simulink model "DCE_motor6_V2"  (R2025a)
settings: Solver=ode4  StartTime=0.0  StopTime=1  FixedStep=5e-5  RelTol=1e-3
undefined symbols (not defined in the file or in its folder): powergui
libraries: spsControlledVoltageSourceLib x24, spsControlledCurrentSourceLib x24, spsVoltageMeasurementLib x24, slpidlib x24, spspowerguiLib x2, simulink x1
(part 2 of 5)

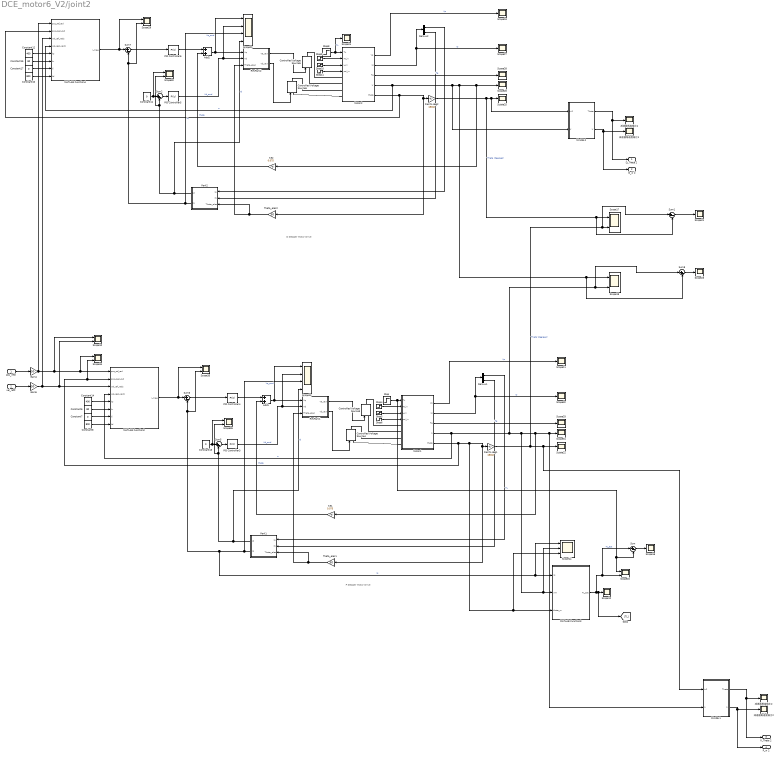
== system DCE_motor6_V2/joint2 ==
  note: D Stepper Motor Drive
  note: P Stepper Motor Drive
  pos_ref2 : Inport
  vel_ref2 : Inport  Port=2
  Add1 : Sum
  Add2 : Sum
  Constant10 : Constant  Value=800
  Constant{7,11,13,17} (4 alike) : Constant  Value=0
  Constant12 : Constant  Value=400
  Constant14 : Constant  Value=400
  Constant15 : Constant  Value=80
  Constant6 : Constant  Value=80
  Constant8 : Constant  Value=800
  Controlled Voltage Source{3..6} (4 alike) : spsControlledVoltageSourceLib/Controlled Voltage Source  Initialize=on  Source_Type=AC  Amplitude=0  Phase=0  Frequency=0  Measurements=None
  Demux1 : Demux  Outputs=2
  Demux2 : Demux  Outputs=2
  Gain4 : Gain  Gain=50
  Gain5 : Gain  Gain=50
  Ke1 : Gain  Gain=0.075
  Ke2 : Gain  Gain=0.075
  MATLAB Function2 : MATLAB Function  TreatAsAtomicUnit=on
  MATLAB Function3 : MATLAB Function  TreatAsAtomicUnit=on
  MATLAB Function4 : MATLAB Function  TreatAsAtomicUnit=on
  Mini08-1 : Subsystem
  Mini08-2 : Subsystem
  Motor1 : Subsystem
  Motor2 : Subsystem
  PID Controller{3..6} (4 alike) : slpidlib/PID Controller  Controller=PI  Form=Parallel  TimeDomain=Discrete-time  UseExternalTs=off  SampleTime=5e-5  IntegratorMethod=Forward Euler  FilterMethod=Forward Euler  ControllerParametersSource=internal  P=5  I=4000  UseKiTs=off  D=0  UseExternalDerivativeSource=off  N=100  UseFilter=on  TunerSelectOption=Transfer Function Based (PID Tuner App)  InitialConditionSource=internal  InitialConditionForIntegrator=0  InitialConditionForFilter=0  DifferentiatorICPrevScaledInput=0  ExternalReset=none  TrackingMode=off  Kt=1  LimitOutput=on  SatLimitsSource=internal  UpperSaturationLimit=24  LowerSaturationLimit=-24  LinearizeAsGain=on  AntiWindupMode=clamping  Kb=1  LimitIntegrator=on  UpperIntegratorSaturationLimit=24  LowerIntegratorSaturationLimit=-24  POutMin=[]  POutMax=[]  IOutMin=[]  IOutMax=[]  DOutMin=[]  DOutMax=[]  NOutMin=[]  NOutMax=[]  SumOutMin=[]  SumOutMax=[]  SaturationOutMin=[]  SaturationOutMax=[]  PParamMin=[]  PParamMax=[]  IParamMin=[]  IParamMax=[]  DParamMin=[]  DParamMax=[]  NParamMin=[]  NParamMax=[]  KbParamMin=[]  KbParamMax=[]  KtParamMin=[]  KtParamMax=[]  KbOutMin=[]  KbOutMax=[]  KtOutMin=[]  KtOutMax=[]  IntegratorOutMin=[]  IntegratorOutMax=[]  FilterOutMin=[]  FilterOutMax=[]  SumI1OutMin=[]  SumI1OutMax=[]  SumI2OutMin=[]  SumI2OutMax=[]  SumI3OutMin=[]  SumI3OutMax=[]  SumI4OutMin=[]  SumI4OutMax=[]  SumDOutMin=[]  SumDOutMax=[]  DifferentiatorOutMin=[]  DifferentiatorOutMax=[]  FilterDiffOutCoefMin=[]  FilterDiffOutCoefMax=[]  ReciprocalOutMin=[]  ReciprocalOutMax=[]  SumDenOutMin=[]  SumDenOutMax=[]  SumNumOutMin=[]  SumNumOutMax=[]  DivideOutMin=[]  DivideOutMax=[]  UdiffTsProdOutMin=[]  UdiffTsProdOutMax=[]  NTsProdOutMin=[]  NTsProdOutMax=[]  UintegralTsProdOutMin=[]  UintegralTsProdOutMax=[]  UngainTsProdOutMin=[]  UngainTsProdOutMax=[]  ClampingZeroOutDataTypeStr=Inherit: Inherit via back propagation  ClampingZeroOutMin=[]  ClampingZeroOutMax=[]  FilterDenConstantOutDataTypeStr=Inherit: Inherit via back propagation  FilterDenConstantOutMin=[]  FilterDenConstantOutMax=[]  PCopyOutDataTypeStr=Inherit: Inherit via back propagation  PCopyOutMin=[]  PCopyOutMax=[]  NCopyOutDataTypeStr=Inherit: Inherit via back propagation  NCopyOutMin=[]  NCopyOutMax=[]  IntegratorContinuousStateAttributes=''  IntegratorStateMustResolveToSignalObject=off  IntegratorRTWStateStorageClass=Auto  FilterContinuousStateAttributes=''  FilterStateMustResolveToSignalObject=off  FilterRTWStateStorageClass=Auto  ParallelPVariant=InternalParameters  IdealPVariant=Disabled  IVariant=InternalParameters  DVariant=Disabled  IntegratorVariant=Discrete  SatVariant=Enabled  AWVariant=DiscClampingParallel  PCopyVariant=Disabled  TRVariant=Disabled  FdbkBlocksVariant=Forward  IdealPFdbkVariant=Disabled  SatFdbkVariant=Disabled  DerivativeFilterVariant=Disabled  NVariant=Disabled  NCopyVariant=Disabled_SignalSpec  FilterICVariant=Disabled  IntegratorICVariant=InternalICs  ExternalResetVariant=Disabled  TRSumVariant=Passthrough  SumFdbkVariant=Disabled  SumVariant=Sum_PI  TsampFilterVariant=InternalTs  TsampNgainVariant=Passthrough  TsampIntegralVariant=Disabled_SignalSpec  ExternalSaturationOutDataTypeStr=Inherit: Same as second input  DerivativeSourceVariant=Disabled  PreIntVariant=InternalPreInt
  Park1 : MATLAB Function  TreatAsAtomicUnit=on
  Park2 : MATLAB Function  TreatAsAtomicUnit=on
  Rad to deg1 : Gain  Gain=180/pi
  Rad to deg2 : Gain  Gain=180/pi
  RevPark1 : MATLAB Function  TreatAsAtomicUnit=on
  RevPark2 : MATLAB Function  TreatAsAtomicUnit=on
  Scope{10,15,17,19,29..30,34..36} (9 alike) : Scope  NumInputPorts=2
      Scope10 settings: ActiveDisplayYMinimum=-5.2481835137744008  ActiveDisplayYMaximum=47.233651623969614  DataLoggingVariableName=ScopeData27
      Scope15 settings: ActiveDisplayYMinimum=0.0075000000000000006  ActiveDisplayYMaximum=0.0325  DataLoggingVariableName=ScopeData34
      Scope17 settings: ActiveDisplayYMinimum=1363.1836491868808  ActiveDisplayYMaximum=1375.04702581976  DataLoggingVariableName=ScopeData36
      Scope19 settings: ActiveDisplayYMinimum=-9.7785388194430141  ActiveDisplayYMaximum=52.407441398347267  DataLoggingVariableName=ScopeData38
      Scope29 settings: ActiveDisplayYMinimum=-0.018504547079538081  ActiveDisplayYMaximum=0.49853620070628168  DataLoggingVariableName=ScopeData28
      Scope30 settings: ActiveDisplayYMinimum=-0.068250226127922337  ActiveDisplayYMaximum=0.064256506451961737  DataLoggingVariableName=ScopeData29
      Scope34 settings: ActiveDisplayYMinimum=-10.860061692792559  ActiveDisplayYMaximum=61.442988659524922  DataLoggingVariableName=ScopeData49
      Scope35 settings: ActiveDisplayYMinimum=-0.018504547079538081  ActiveDisplayYMaximum=0.49853620070628168  DataLoggingVariableName=ScopeData50
      Scope36 settings: ActiveDisplayYMinimum=-0.068250226127922337  ActiveDisplayYMaximum=0.064256506451961737  DataLoggingVariableName=ScopeData51
  Scope{11..12,16,18,21..28,31..33} (15 alike) : Scope
      Scope11 settings: ActiveDisplayYMinimum=-19.096901402816375  ActiveDisplayYMaximum=19.120590576315788  DataLoggingVariableName=ScopeData30
      Scope12 settings: ActiveDisplayYMinimum=0.0055558714492785766  ActiveDisplayYMaximum=0.04791549784383016  DataLoggingVariableName=ScopeData31
      Scope16 settings: ActiveDisplayYMinimum=-0.00045623090907525666  ActiveDisplayYMaximum=0.00044225246132360179  DataLoggingVariableName=ScopeData35
      Scope18 settings: ActiveDisplayYMinimum=-19.096901402816375  ActiveDisplayYMaximum=19.120590576315788  DataLoggingVariableName=ScopeData37
      Scope21 settings: ActiveDisplayYMinimum=-9.08103109878298  ActiveDisplayYMaximum=1.6684669955642857  DataLoggingVariableName=ScopeData40
      Scope22 settings: ActiveDisplayYMinimum=-70.559876705932709  ActiveDisplayYMaximum=631.53921004933659  DataLoggingVariableName=ScopeData41
      Scope23 settings: ActiveDisplayYMinimum=-1.5635296954169715  ActiveDisplayYMaximum=0.72593411203052016  DataLoggingVariableName=ScopeData42
      Scope24 settings: ActiveDisplayYMinimum=-0.0062150346375224163  ActiveDisplayYMaximum=0.055935311737701762  DataLoggingVariableName=ScopeData43
      Scope25 settings: ActiveDisplayYMinimum=-70.559876705932709  ActiveDisplayYMaximum=631.53921004933659  DataLoggingVariableName=ScopeData44
      Scope26 settings: ActiveDisplayYMinimum=-452.6835395386438  ActiveDisplayYMaximum=318.93705127381384  DataLoggingVariableName=ScopeData45
      Scope27 settings: ActiveDisplayYMinimum=-0.40449771436693455  ActiveDisplayYMaximum=0.64067173662257559  DataLoggingVariableName=ScopeData25
      Scope28 settings: ActiveDisplayYMinimum=-0.046646220623980633  ActiveDisplayYMaximum=0.10063848186154864  DataLoggingVariableName=ScopeData26
      Scope31 settings: ActiveDisplayYMinimum=-115.17645332437448  ActiveDisplayYMaximum=118.37044346456712  DataLoggingVariableName=ScopeData46
      Scope32 settings: ActiveDisplayYMinimum=-0.40449771436693455  ActiveDisplayYMaximum=0.64067173662257559  DataLoggingVariableName=ScopeData47
      Scope33 settings: ActiveDisplayYMinimum=-0.046646220623980633  ActiveDisplayYMaximum=0.10063848186154864  DataLoggingVariableName=ScopeData48
  Scope13 : Scope  NumInputPorts=4
      settings: ActiveDisplayYMinimum=-0.68813129304418319  ActiveDisplayYMaximum=6.2555990509558841  DataLoggingVariableName=ScopeData32
  Scope14 : Scope  NumInputPorts=3
      settings: ActiveDisplayYMinimum=-0.052783691584462819  ActiveDisplayYMaximum=0.4750532242601655  DataLoggingVariableName=ScopeData33
  Scope20 : Scope  NumInputPorts=4
      settings: ActiveDisplayYMinimum=-0.68813129304418319  ActiveDisplayYMaximum=6.2555990509558841  DataLoggingVariableName=ScopeData39
  Step : Step  Time=0  Before=0.01  After=0.01  SampleTime=0
  Step10 : Step  Time=0  Before=0.00544  After=0.00544  SampleTime=0
  Step11 : Step  Time=0  Before=0.0015  After=0.0015  SampleTime=0
  Step4 : Step  Time=0  Before=4.85  After=4.85  SampleTime=0
  Step5 : Step  Time=0  Before=0.00544  After=0.00544  SampleTime=0
  Step6 : Step  Time=0  Before=0.0015  After=0.0015  SampleTime=0
  Step8 : Step  Time=0  Before=0.01  After=0.01  SampleTime=0
  Step9 : Step  Time=0  Before=4.85  After=4.85  SampleTime=0
  Sum{,1..2,5..8} (7 alike) : Sum  Inputs=|+-
  Theta_elec1 : Gain  Gain=50
  Theta_elec2 : Gain  Gain=50
  减速器角度输出1 : Scope
      settings: ActiveDisplayYMinimum=-3.2575204385667078  ActiveDisplayYMaximum=25.318176358378867  DataLoggingVariableName=ScopeData53
  减速器角度输出2 : Scope
      settings: ActiveDisplayYMinimum=-3.2575204385667078  ActiveDisplayYMaximum=25.318176358378867  DataLoggingVariableName=ScopeData56
  减速器角速度输出1 : Scope
      settings: ActiveDisplayYMinimum=-0.049701649268213327  ActiveDisplayYMaximum=0.44324985732957672  DataLoggingVariableName=ScopeData54
  减速器角速度输出2 : Scope
      settings: ActiveDisplayYMinimum=-0.049701649268213327  ActiveDisplayYMaximum=0.44324985732957672  DataLoggingVariableName=ScopeData57
  D_Theta 2 : Outport
  D_w 2 : Outport  Port=2
  P_Theta 2 : Outport  Port=3
  P_w 2 : Outport  Port=4
  wires:
  Sum8/1 -> Scope23/1
  Sum1/1 -> Scope21/1
  Step8/1 -> Scope24/1, Motor2/1(TL)  "TL"
  Motor2/1(Vp) -> Scope18/1  "Vp"
  Motor2/2(Ip) -> Demux2/1, Scope27/1  "Ip"
  Park2/2(Iq) -> Scope20/3, Scope29/2, Sum7/2  "Iq"
  Park2/1(Id) -> Scope20/4, Scope30/2, Sum2/2  "Id"
  Constant11/1 -> Scope30/1, Sum2/1
  PID Controller6/1 -> Add2/1
  MATLAB Function4/1(I_mag) -> Scope29/1, Sum7/1
  Demux2/1 -> Park2/1(Ia)
  Sum7/1 -> PID Controller6/1
  Motor2/5(theta) -> MATLAB Function4/2(pos_real_rad), Rad to deg2/1, Theta_elec2/1  "theta"
  Constant12/1 -> MATLAB Function4/5(kp)
  Sum2/1 -> PID Controller5/1
  Step10/1 -> Motor2/3(L_in)
  Ke2/1 -> Add2/2
  Motor2/3(Te) -> Scope28/1  "Te"
  RevPark2/2(Vb_raw) -> Controlled Voltage Source6/1
  Step11/1 -> Motor2/4(psi_in)
  Theta_elec2/1 -> RevPark2/3(Theta_elec), Park2/3(Theta_elec)
  Constant17/1 -> MATLAB Function4/7(ki)
  Add2/1 -> Scope20/1, RevPark2/1(Vq)  "Vq_cmd"
  PID Controller5/1 -> Scope20/2, RevPark2/2(Vd)  "Vd_cmd"
  Step/1 -> Sum/2, Scope15/1, Motor1/1(TL)  "TL"
  Motor2/4(w) -> MATLAB Function4/4(vel_real_rads), Mini08-2/2(w), Sum8/2, Scope19/1, Ke2/1, Scope26/1  "w"
  MATLAB Function3/1(TL_est) -> Sum/1, Scope15/2, [TL], Scope12/1  "TL_est"
  Sum/1 -> Scope16/1
  PID Controller3/1 -> Scope13/2, RevPark1/2(Vd)  "Vd_cmd"
  Motor1/4(w) -> MATLAB Function2/4(vel_real_rads), Sum8/1, Scope19/2, Scope14/2, MATLAB Function3/2(wm), Ke1/1, Mini08-1/2(w), Scope31/1  "w"
  Step9/1 -> Motor2/2(IR_in)
  Add1/1 -> Scope13/1, RevPark1/1(Vq)  "Vq_cmd"
  Constant14/1 -> MATLAB Function2/5(kp)
  Park1/1(Id) -> Scope13/4, Scope36/2, Sum5/2  "Id"
  Constant6/1 -> MATLAB Function2/6(kv)
  Constant15/1 -> MATLAB Function4/6(kv)
  Constant7/1 -> MATLAB Function2/7(ki)
  Theta_elec1/1 -> RevPark1/3(Theta_elec), Park1/3(Theta_elec)
  Motor1/5(theta) -> Scope34/2, MATLAB Function2/2(pos_real_rad), Scope14/3, MATLAB Function3/3(theta_m), Rad to deg1/1, Theta_elec1/1  "theta"
  Sum5/1 -> PID Controller3/1
  Step5/1 -> Motor1/3(L_in)
  Ke1/1 -> Add1/2
  Step6/1 -> Motor1/4(psi_in)
  Sum6/1 -> PID Controller4/1
  Rad to deg1/1 -> Sum1/1, Scope17/2, Mini08-1/1(In2), Scope22/1  "Theta (degrees)"
  RevPark1/2(Vb_raw) -> Controlled Voltage Source4/1
  Demux2/2 -> Park2/2(Ib)
  Motor1/3(Te) -> Scope33/1  "Te"
  Rad to deg2/1 -> Sum1/2, Scope17/1, Mini08-2/1(In2), Scope25/1  "Theta (degrees)"
  RevPark1/1(Va_raw) -> Controlled Voltage Source3/1
  Constant8/1 -> MATLAB Function2/8(kd)
  Demux1/1 -> Park1/1(Ia)
  Motor1/1(Vp) -> Scope11/1  "Vp"
  RevPark2/1(Va_raw) -> Controlled Voltage Source5/1
  Step4/1 -> Motor1/2(IR_in)
  Park1/2(Iq) -> Scope13/3, Scope14/1, MATLAB Function3/1(iq), Scope35/2, Sum6/2  "Iq"
  Constant10/1 -> MATLAB Function4/8(kd)
  MATLAB Function2/1(I_mag) -> Scope35/1, Sum6/1
  Motor1/2(Ip) -> Demux1/1, Scope32/1  "Ip"
  Constant13/1 -> Scope36/1, Sum5/1
  PID Controller4/1 -> Add1/1
  Demux1/2 -> Park1/2(Ib)
  vel_ref2/1 -> Gain5/1
  Gain4/1 -> Scope10/1, Scope34/1, MATLAB Function2/1(pos_ref_rad), MATLAB Function4/1(pos_ref_rad)
  pos_ref2/1 -> Gain4/1
  Gain5/1 -> Scope10/2, MATLAB Function2/3(vel_ref_rads), MATLAB Function4/3(vel_ref_rads)
  Mini08-2/1("Theta ") -> D_Theta 2/1, 减速器角度输出1/1
  Mini08-2/2("w ") -> D_w 2/1, 减速器角速度输出1/1
  Mini08-1/2("w ") -> P_w 2/1, 减速器角速度输出2/1
  Mini08-1/1("Theta ") -> P_Theta 2/1, 减速器角度输出2/1
  connections:
  Motor1/LConn4 -- Controlled Voltage Source4/LConn1
  Motor2/LConn4 -- Controlled Voltage Source6/LConn1
  Motor1/LConn2 -- Controlled Voltage Source3/LConn1
  Motor2/LConn1 -- Controlled Voltage Source5/RConn1
  Motor1/LConn1 -- Controlled Voltage Source3/RConn1
  Motor2/LConn2 -- Controlled Voltage Source5/LConn1
  Motor1/LConn3 -- Controlled Voltage Source4/RConn1
  Motor2/LConn3 -- Controlled Voltage Source6/RConn1

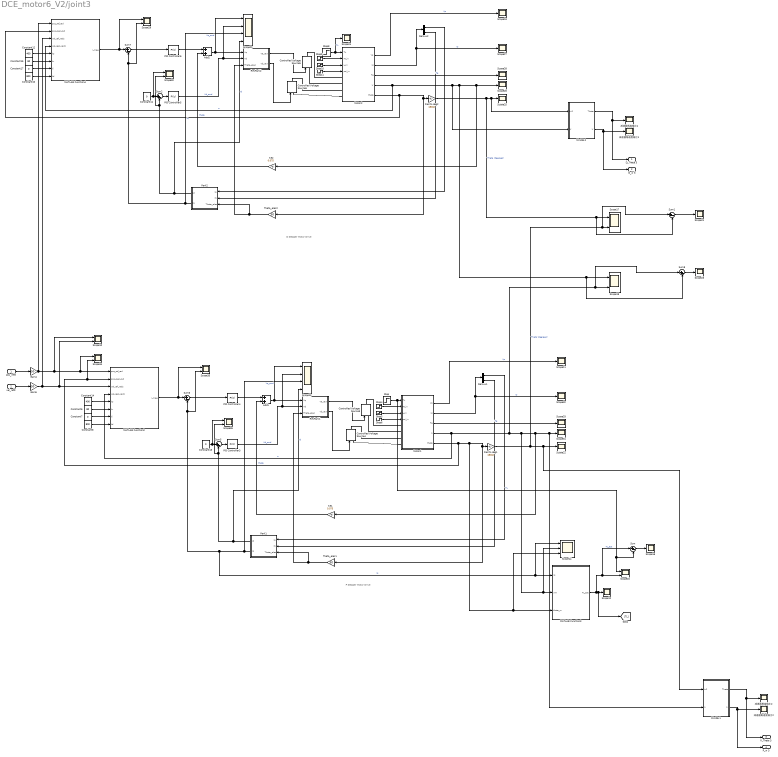
== system DCE_motor6_V2/joint3 ==
  note: D Stepper Motor Drive
  note: P Stepper Motor Drive
  pos_ref3 : Inport
  vel_ref3 : Inport  Port=2
  Add1 : Sum
  Add2 : Sum
  Constant10 : Constant  Value=800
  Constant{7,11,13,17} (4 alike) : Constant  Value=0
  Constant12 : Constant  Value=400
  Constant14 : Constant  Value=400
  Constant15 : Constant  Value=80
  Constant6 : Constant  Value=80
  Constant8 : Constant  Value=800
  Controlled Voltage Source{3..6} (4 alike) : spsControlledVoltageSourceLib/Controlled Voltage Source  Initialize=on  Source_Type=AC  Amplitude=0  Phase=0  Frequency=0  Measurements=None
  Demux1 : Demux  Outputs=2
  Demux2 : Demux  Outputs=2
  Gain4 : Gain  Gain=50
  Gain5 : Gain  Gain=50
  Ke1 : Gain  Gain=0.075
  Ke2 : Gain  Gain=0.075
  MATLAB Function2 : MATLAB Function  TreatAsAtomicUnit=on
  MATLAB Function3 : MATLAB Function  TreatAsAtomicUnit=on
  MATLAB Function4 : MATLAB Function  TreatAsAtomicUnit=on
  Mini08-1 : Subsystem
  Mini08-2 : Subsystem
  Motor1 : Subsystem
  Motor2 : Subsystem
  PID Controller{3..6} (4 alike) : slpidlib/PID Controller  Controller=PI  Form=Parallel  TimeDomain=Discrete-time  UseExternalTs=off  SampleTime=5e-5  IntegratorMethod=Forward Euler  FilterMethod=Forward Euler  ControllerParametersSource=internal  P=5  I=4000  UseKiTs=off  D=0  UseExternalDerivativeSource=off  N=100  UseFilter=on  TunerSelectOption=Transfer Function Based (PID Tuner App)  InitialConditionSource=internal  InitialConditionForIntegrator=0  InitialConditionForFilter=0  DifferentiatorICPrevScaledInput=0  ExternalReset=none  TrackingMode=off  Kt=1  LimitOutput=on  SatLimitsSource=internal  UpperSaturationLimit=24  LowerSaturationLimit=-24  LinearizeAsGain=on  AntiWindupMode=clamping  Kb=1  LimitIntegrator=on  UpperIntegratorSaturationLimit=24  LowerIntegratorSaturationLimit=-24  POutMin=[]  POutMax=[]  IOutMin=[]  IOutMax=[]  DOutMin=[]  DOutMax=[]  NOutMin=[]  NOutMax=[]  SumOutMin=[]  SumOutMax=[]  SaturationOutMin=[]  SaturationOutMax=[]  PParamMin=[]  PParamMax=[]  IParamMin=[]  IParamMax=[]  DParamMin=[]  DParamMax=[]  NParamMin=[]  NParamMax=[]  KbParamMin=[]  KbParamMax=[]  KtParamMin=[]  KtParamMax=[]  KbOutMin=[]  KbOutMax=[]  KtOutMin=[]  KtOutMax=[]  IntegratorOutMin=[]  IntegratorOutMax=[]  FilterOutMin=[]  FilterOutMax=[]  SumI1OutMin=[]  SumI1OutMax=[]  SumI2OutMin=[]  SumI2OutMax=[]  SumI3OutMin=[]  SumI3OutMax=[]  SumI4OutMin=[]  SumI4OutMax=[]  SumDOutMin=[]  SumDOutMax=[]  DifferentiatorOutMin=[]  DifferentiatorOutMax=[]  FilterDiffOutCoefMin=[]  FilterDiffOutCoefMax=[]  ReciprocalOutMin=[]  ReciprocalOutMax=[]  SumDenOutMin=[]  SumDenOutMax=[]  SumNumOutMin=[]  SumNumOutMax=[]  DivideOutMin=[]  DivideOutMax=[]  UdiffTsProdOutMin=[]  UdiffTsProdOutMax=[]  NTsProdOutMin=[]  NTsProdOutMax=[]  UintegralTsProdOutMin=[]  UintegralTsProdOutMax=[]  UngainTsProdOutMin=[]  UngainTsProdOutMax=[]  ClampingZeroOutDataTypeStr=Inherit: Inherit via back propagation  ClampingZeroOutMin=[]  ClampingZeroOutMax=[]  FilterDenConstantOutDataTypeStr=Inherit: Inherit via back propagation  FilterDenConstantOutMin=[]  FilterDenConstantOutMax=[]  PCopyOutDataTypeStr=Inherit: Inherit via back propagation  PCopyOutMin=[]  PCopyOutMax=[]  NCopyOutDataTypeStr=Inherit: Inherit via back propagation  NCopyOutMin=[]  NCopyOutMax=[]  IntegratorContinuousStateAttributes=''  IntegratorStateMustResolveToSignalObject=off  IntegratorRTWStateStorageClass=Auto  FilterContinuousStateAttributes=''  FilterStateMustResolveToSignalObject=off  FilterRTWStateStorageClass=Auto  ParallelPVariant=InternalParameters  IdealPVariant=Disabled  IVariant=InternalParameters  DVariant=Disabled  IntegratorVariant=Discrete  SatVariant=Enabled  AWVariant=DiscClampingParallel  PCopyVariant=Disabled  TRVariant=Disabled  FdbkBlocksVariant=Forward  IdealPFdbkVariant=Disabled  SatFdbkVariant=Disabled  DerivativeFilterVariant=Disabled  NVariant=Disabled  NCopyVariant=Disabled_SignalSpec  FilterICVariant=Disabled  IntegratorICVariant=InternalICs  ExternalResetVariant=Disabled  TRSumVariant=Passthrough  SumFdbkVariant=Disabled  SumVariant=Sum_PI  TsampFilterVariant=InternalTs  TsampNgainVariant=Passthrough  TsampIntegralVariant=Disabled_SignalSpec  ExternalSaturationOutDataTypeStr=Inherit: Same as second input  DerivativeSourceVariant=Disabled  PreIntVariant=InternalPreInt
  Park1 : MATLAB Function  TreatAsAtomicUnit=on
  Park2 : MATLAB Function  TreatAsAtomicUnit=on
  Rad to deg1 : Gain  Gain=180/pi
  Rad to deg2 : Gain  Gain=180/pi
  RevPark1 : MATLAB Function  TreatAsAtomicUnit=on
  RevPark2 : MATLAB Function  TreatAsAtomicUnit=on
  Scope{10,15,17,19,29..30,34..36} (9 alike) : Scope  NumInputPorts=2
      Scope10 settings: ActiveDisplayYMinimum=-5.2481835137744008  ActiveDisplayYMaximum=47.233651623969614  DataLoggingVariableName=ScopeData27
      Scope15 settings: ActiveDisplayYMinimum=0.0075000000000000006  ActiveDisplayYMaximum=0.0325  DataLoggingVariableName=ScopeData34
      Scope17 settings: ActiveDisplayYMinimum=1363.1836491868808  ActiveDisplayYMaximum=1375.04702581976  DataLoggingVariableName=ScopeData36
      Scope19 settings: ActiveDisplayYMinimum=-9.7785388194430141  ActiveDisplayYMaximum=52.407441398347267  DataLoggingVariableName=ScopeData38
      Scope29 settings: ActiveDisplayYMinimum=-0.018504547079538081  ActiveDisplayYMaximum=0.49853620070628168  DataLoggingVariableName=ScopeData28
      Scope30 settings: ActiveDisplayYMinimum=-0.068250226127922337  ActiveDisplayYMaximum=0.064256506451961737  DataLoggingVariableName=ScopeData29
      Scope34 settings: ActiveDisplayYMinimum=-10.860061692792559  ActiveDisplayYMaximum=61.442988659524922  DataLoggingVariableName=ScopeData49
      Scope35 settings: ActiveDisplayYMinimum=-0.018504547079538081  ActiveDisplayYMaximum=0.49853620070628168  DataLoggingVariableName=ScopeData50
      Scope36 settings: ActiveDisplayYMinimum=-0.068250226127922337  ActiveDisplayYMaximum=0.064256506451961737  DataLoggingVariableName=ScopeData51
  Scope{11..12,16,18,21..28,31..33} (15 alike) : Scope
      Scope11 settings: ActiveDisplayYMinimum=-19.096901402816375  ActiveDisplayYMaximum=19.120590576315788  DataLoggingVariableName=ScopeData30
      Scope12 settings: ActiveDisplayYMinimum=0.0055558714492785766  ActiveDisplayYMaximum=0.04791549784383016  DataLoggingVariableName=ScopeData31
      Scope16 settings: ActiveDisplayYMinimum=-0.00045623090907525666  ActiveDisplayYMaximum=0.00044225246132360179  DataLoggingVariableName=ScopeData35
      Scope18 settings: ActiveDisplayYMinimum=-19.096901402816375  ActiveDisplayYMaximum=19.120590576315788  DataLoggingVariableName=ScopeData37
      Scope21 settings: ActiveDisplayYMinimum=-9.08103109878298  ActiveDisplayYMaximum=1.6684669955642857  DataLoggingVariableName=ScopeData40
      Scope22 settings: ActiveDisplayYMinimum=-70.559876705932709  ActiveDisplayYMaximum=631.53921004933659  DataLoggingVariableName=ScopeData41
      Scope23 settings: ActiveDisplayYMinimum=-1.5635296954169715  ActiveDisplayYMaximum=0.72593411203052016  DataLoggingVariableName=ScopeData42
      Scope24 settings: ActiveDisplayYMinimum=-0.0062150346375224163  ActiveDisplayYMaximum=0.055935311737701762  DataLoggingVariableName=ScopeData43
      Scope25 settings: ActiveDisplayYMinimum=-70.559876705932709  ActiveDisplayYMaximum=631.53921004933659  DataLoggingVariableName=ScopeData44
      Scope26 settings: ActiveDisplayYMinimum=-452.6835395386438  ActiveDisplayYMaximum=318.93705127381384  DataLoggingVariableName=ScopeData45
      Scope27 settings: ActiveDisplayYMinimum=-0.40449771436693455  ActiveDisplayYMaximum=0.64067173662257559  DataLoggingVariableName=ScopeData25
      Scope28 settings: ActiveDisplayYMinimum=-0.046646220623980633  ActiveDisplayYMaximum=0.10063848186154864  DataLoggingVariableName=ScopeData26
      Scope31 settings: ActiveDisplayYMinimum=-115.17645332437448  ActiveDisplayYMaximum=118.37044346456712  DataLoggingVariableName=ScopeData46
      Scope32 settings: ActiveDisplayYMinimum=-0.40449771436693455  ActiveDisplayYMaximum=0.64067173662257559  DataLoggingVariableName=ScopeData47
      Scope33 settings: ActiveDisplayYMinimum=-0.046646220623980633  ActiveDisplayYMaximum=0.10063848186154864  DataLoggingVariableName=ScopeData48
  Scope13 : Scope  NumInputPorts=4
      settings: ActiveDisplayYMinimum=-0.68813129304418319  ActiveDisplayYMaximum=6.2555990509558841  DataLoggingVariableName=ScopeData32
  Scope14 : Scope  NumInputPorts=3
      settings: ActiveDisplayYMinimum=-0.052783691584462819  ActiveDisplayYMaximum=0.4750532242601655  DataLoggingVariableName=ScopeData33
  Scope20 : Scope  NumInputPorts=4
      settings: ActiveDisplayYMinimum=-0.68813129304418319  ActiveDisplayYMaximum=6.2555990509558841  DataLoggingVariableName=ScopeData39
  Step : Step  Time=0  Before=0.01  After=0.01  SampleTime=0
  Step10 : Step  Time=0  Before=0.00544  After=0.00544  SampleTime=0
  Step11 : Step  Time=0  Before=0.0015  After=0.0015  SampleTime=0
  Step4 : Step  Time=0  Before=4.85  After=4.85  SampleTime=0
  Step5 : Step  Time=0  Before=0.00544  After=0.00544  SampleTime=0
  Step6 : Step  Time=0  Before=0.0015  After=0.0015  SampleTime=0
  Step8 : Step  Time=0  Before=0.01  After=0.01  SampleTime=0
  Step9 : Step  Time=0  Before=4.85  After=4.85  SampleTime=0
  Sum{,1..2,5..8} (7 alike) : Sum  Inputs=|+-
  Theta_elec1 : Gain  Gain=50
  Theta_elec2 : Gain  Gain=50
  减速器角度输出1 : Scope
      settings: ActiveDisplayYMinimum=-3.2575204385667078  ActiveDisplayYMaximum=25.318176358378867  DataLoggingVariableName=ScopeData53
  减速器角度输出2 : Scope
      settings: ActiveDisplayYMinimum=-3.2575204385667078  ActiveDisplayYMaximum=25.318176358378867  DataLoggingVariableName=ScopeData56
  减速器角速度输出1 : Scope
      settings: ActiveDisplayYMinimum=-0.049701649268213327  ActiveDisplayYMaximum=0.44324985732957672  DataLoggingVariableName=ScopeData54
  减速器角速度输出2 : Scope
      settings: ActiveDisplayYMinimum=-0.049701649268213327  ActiveDisplayYMaximum=0.44324985732957672  DataLoggingVariableName=ScopeData57
  D_Theta 3 : Outport
  D_w 3 : Outport  Port=2
  P_Theta 3 : Outport  Port=3
  P_w 3 : Outport  Port=4
  wires:
  Sum8/1 -> Scope23/1
  Sum1/1 -> Scope21/1
  Step8/1 -> Scope24/1, Motor2/1(TL)  "TL"
  Motor2/1(Vp) -> Scope18/1  "Vp"
  Motor2/2(Ip) -> Demux2/1, Scope27/1  "Ip"
  Park2/2(Iq) -> Scope20/3, Scope29/2, Sum7/2  "Iq"
  Park2/1(Id) -> Scope20/4, Scope30/2, Sum2/2  "Id"
  Constant11/1 -> Scope30/1, Sum2/1
  PID Controller6/1 -> Add2/1
  MATLAB Function4/1(I_mag) -> Scope29/1, Sum7/1
  Demux2/1 -> Park2/1(Ia)
  Sum7/1 -> PID Controller6/1
  Motor2/5(theta) -> MATLAB Function4/2(pos_real_rad), Rad to deg2/1, Theta_elec2/1  "theta"
  Constant12/1 -> MATLAB Function4/5(kp)
  Sum2/1 -> PID Controller5/1
  Step10/1 -> Motor2/3(L_in)
  Ke2/1 -> Add2/2
  Motor2/3(Te) -> Scope28/1  "Te"
  RevPark2/2(Vb_raw) -> Controlled Voltage Source6/1
  Step11/1 -> Motor2/4(psi_in)
  Theta_elec2/1 -> RevPark2/3(Theta_elec), Park2/3(Theta_elec)
  Constant17/1 -> MATLAB Function4/7(ki)
  Add2/1 -> Scope20/1, RevPark2/1(Vq)  "Vq_cmd"
  PID Controller5/1 -> Scope20/2, RevPark2/2(Vd)  "Vd_cmd"
  Step/1 -> Sum/2, Scope15/1, Motor1/1(TL)  "TL"
  Motor2/4(w) -> MATLAB Function4/4(vel_real_rads), Mini08-2/2(w), Sum8/2, Scope19/1, Ke2/1, Scope26/1  "w"
  MATLAB Function3/1(TL_est) -> Sum/1, Scope15/2, [TL], Scope12/1  "TL_est"
  Sum/1 -> Scope16/1
  PID Controller3/1 -> Scope13/2, RevPark1/2(Vd)  "Vd_cmd"
  Motor1/4(w) -> MATLAB Function2/4(vel_real_rads), Sum8/1, Scope19/2, Scope14/2, MATLAB Function3/2(wm), Ke1/1, Mini08-1/2(w), Scope31/1  "w"
  Step9/1 -> Motor2/2(IR_in)
  Add1/1 -> Scope13/1, RevPark1/1(Vq)  "Vq_cmd"
  Constant14/1 -> MATLAB Function2/5(kp)
  Park1/1(Id) -> Scope13/4, Scope36/2, Sum5/2  "Id"
  Constant6/1 -> MATLAB Function2/6(kv)
  Constant15/1 -> MATLAB Function4/6(kv)
  Constant7/1 -> MATLAB Function2/7(ki)
  Theta_elec1/1 -> RevPark1/3(Theta_elec), Park1/3(Theta_elec)
  Motor1/5(theta) -> Scope34/2, MATLAB Function2/2(pos_real_rad), Scope14/3, MATLAB Function3/3(theta_m), Rad to deg1/1, Theta_elec1/1  "theta"
  Sum5/1 -> PID Controller3/1
  Step5/1 -> Motor1/3(L_in)
  Ke1/1 -> Add1/2
  Step6/1 -> Motor1/4(psi_in)
  Sum6/1 -> PID Controller4/1
  Rad to deg1/1 -> Sum1/1, Scope17/2, Mini08-1/1(In2), Scope22/1  "Theta (degrees)"
  RevPark1/2(Vb_raw) -> Controlled Voltage Source4/1
  Demux2/2 -> Park2/2(Ib)
  Motor1/3(Te) -> Scope33/1  "Te"
  Rad to deg2/1 -> Sum1/2, Scope17/1, Mini08-2/1(In2), Scope25/1  "Theta (degrees)"
  RevPark1/1(Va_raw) -> Controlled Voltage Source3/1
  Constant8/1 -> MATLAB Function2/8(kd)
  Demux1/1 -> Park1/1(Ia)
  Motor1/1(Vp) -> Scope11/1  "Vp"
  RevPark2/1(Va_raw) -> Controlled Voltage Source5/1
  Step4/1 -> Motor1/2(IR_in)
  Park1/2(Iq) -> Scope13/3, Scope14/1, MATLAB Function3/1(iq), Scope35/2, Sum6/2  "Iq"
  Constant10/1 -> MATLAB Function4/8(kd)
  MATLAB Function2/1(I_mag) -> Scope35/1, Sum6/1
  Motor1/2(Ip) -> Demux1/1, Scope32/1  "Ip"
  Constant13/1 -> Scope36/1, Sum5/1
  PID Controller4/1 -> Add1/1
  Demux1/2 -> Park1/2(Ib)
  vel_ref3/1 -> Gain5/1
  Gain4/1 -> Scope10/1, Scope34/1, MATLAB Function2/1(pos_ref_rad), MATLAB Function4/1(pos_ref_rad)
  pos_ref3/1 -> Gain4/1
  Gain5/1 -> Scope10/2, MATLAB Function2/3(vel_ref_rads), MATLAB Function4/3(vel_ref_rads)
  Mini08-2/1("Theta ") -> D_Theta 3/1, 减速器角度输出1/1
  Mini08-2/2("w ") -> D_w 3/1, 减速器角速度输出1/1
  Mini08-1/2("w ") -> P_w 3/1, 减速器角速度输出2/1
  Mini08-1/1("Theta ") -> P_Theta 3/1, 减速器角度输出2/1
  connections:
  Motor1/LConn4 -- Controlled Voltage Source4/LConn1
  Motor2/LConn4 -- Controlled Voltage Source6/LConn1
  Motor1/LConn2 -- Controlled Voltage Source3/LConn1
  Motor2/LConn1 -- Controlled Voltage Source5/RConn1
  Motor1/LConn1 -- Controlled Voltage Source3/RConn1
  Motor2/LConn2 -- Controlled Voltage Source5/LConn1
  Motor1/LConn3 -- Controlled Voltage Source4/RConn1
  Motor2/LConn3 -- Controlled Voltage Source6/RConn1

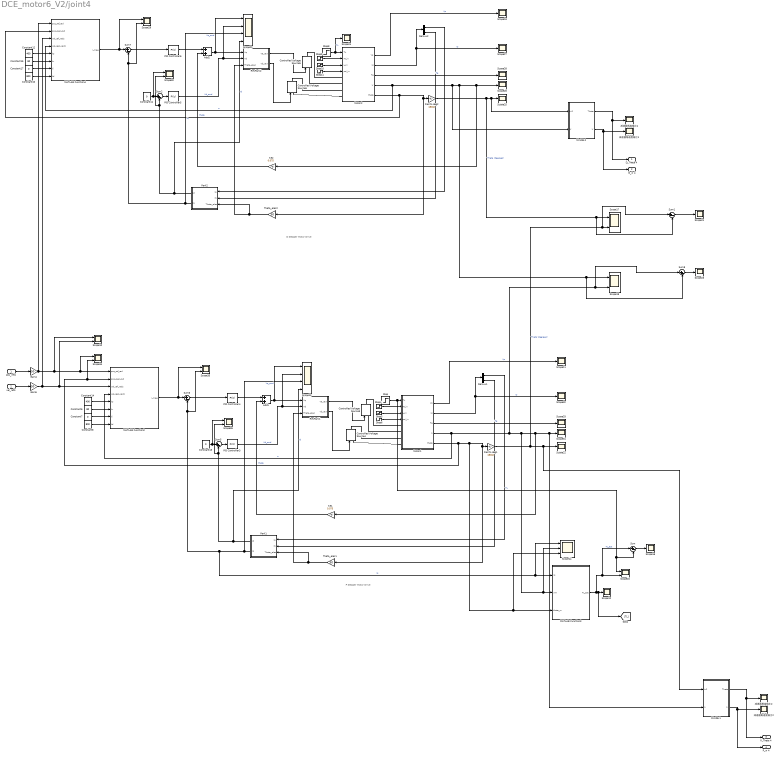
== system DCE_motor6_V2/joint4 ==
  note: D Stepper Motor Drive
  note: P Stepper Motor Drive
  pos_ref4 : Inport
  vel_ref4 : Inport  Port=2
  Add1 : Sum
  Add2 : Sum
  Constant10 : Constant  Value=800
  Constant{7,11,13,17} (4 alike) : Constant  Value=0
  Constant12 : Constant  Value=400
  Constant14 : Constant  Value=400
  Constant15 : Constant  Value=80
  Constant6 : Constant  Value=80
  Constant8 : Constant  Value=800
  Controlled Voltage Source{3..6} (4 alike) : spsControlledVoltageSourceLib/Controlled Voltage Source  Initialize=on  Source_Type=AC  Amplitude=0  Phase=0  Frequency=0  Measurements=None
  Demux1 : Demux  Outputs=2
  Demux2 : Demux  Outputs=2
  Gain4 : Gain  Gain=50
  Gain5 : Gain  Gain=50
  Ke1 : Gain  Gain=0.075
  Ke2 : Gain  Gain=0.075
  MATLAB Function2 : MATLAB Function  TreatAsAtomicUnit=on
  MATLAB Function3 : MATLAB Function  TreatAsAtomicUnit=on
  MATLAB Function4 : MATLAB Function  TreatAsAtomicUnit=on
  Mini08-1 : Subsystem
  Mini08-2 : Subsystem
  Motor1 : Subsystem
  Motor2 : Subsystem
  PID Controller{3..6} (4 alike) : slpidlib/PID Controller  Controller=PI  Form=Parallel  TimeDomain=Discrete-time  UseExternalTs=off  SampleTime=5e-5  IntegratorMethod=Forward Euler  FilterMethod=Forward Euler  ControllerParametersSource=internal  P=5  I=4000  UseKiTs=off  D=0  UseExternalDerivativeSource=off  N=100  UseFilter=on  TunerSelectOption=Transfer Function Based (PID Tuner App)  InitialConditionSource=internal  InitialConditionForIntegrator=0  InitialConditionForFilter=0  DifferentiatorICPrevScaledInput=0  ExternalReset=none  TrackingMode=off  Kt=1  LimitOutput=on  SatLimitsSource=internal  UpperSaturationLimit=24  LowerSaturationLimit=-24  LinearizeAsGain=on  AntiWindupMode=clamping  Kb=1  LimitIntegrator=on  UpperIntegratorSaturationLimit=24  LowerIntegratorSaturationLimit=-24  POutMin=[]  POutMax=[]  IOutMin=[]  IOutMax=[]  DOutMin=[]  DOutMax=[]  NOutMin=[]  NOutMax=[]  SumOutMin=[]  SumOutMax=[]  SaturationOutMin=[]  SaturationOutMax=[]  PParamMin=[]  PParamMax=[]  IParamMin=[]  IParamMax=[]  DParamMin=[]  DParamMax=[]  NParamMin=[]  NParamMax=[]  KbParamMin=[]  KbParamMax=[]  KtParamMin=[]  KtParamMax=[]  KbOutMin=[]  KbOutMax=[]  KtOutMin=[]  KtOutMax=[]  IntegratorOutMin=[]  IntegratorOutMax=[]  FilterOutMin=[]  FilterOutMax=[]  SumI1OutMin=[]  SumI1OutMax=[]  SumI2OutMin=[]  SumI2OutMax=[]  SumI3OutMin=[]  SumI3OutMax=[]  SumI4OutMin=[]  SumI4OutMax=[]  SumDOutMin=[]  SumDOutMax=[]  DifferentiatorOutMin=[]  DifferentiatorOutMax=[]  FilterDiffOutCoefMin=[]  FilterDiffOutCoefMax=[]  ReciprocalOutMin=[]  ReciprocalOutMax=[]  SumDenOutMin=[]  SumDenOutMax=[]  SumNumOutMin=[]  SumNumOutMax=[]  DivideOutMin=[]  DivideOutMax=[]  UdiffTsProdOutMin=[]  UdiffTsProdOutMax=[]  NTsProdOutMin=[]  NTsProdOutMax=[]  UintegralTsProdOutMin=[]  UintegralTsProdOutMax=[]  UngainTsProdOutMin=[]  UngainTsProdOutMax=[]  ClampingZeroOutDataTypeStr=Inherit: Inherit via back propagation  ClampingZeroOutMin=[]  ClampingZeroOutMax=[]  FilterDenConstantOutDataTypeStr=Inherit: Inherit via back propagation  FilterDenConstantOutMin=[]  FilterDenConstantOutMax=[]  PCopyOutDataTypeStr=Inherit: Inherit via back propagation  PCopyOutMin=[]  PCopyOutMax=[]  NCopyOutDataTypeStr=Inherit: Inherit via back propagation  NCopyOutMin=[]  NCopyOutMax=[]  IntegratorContinuousStateAttributes=''  IntegratorStateMustResolveToSignalObject=off  IntegratorRTWStateStorageClass=Auto  FilterContinuousStateAttributes=''  FilterStateMustResolveToSignalObject=off  FilterRTWStateStorageClass=Auto  ParallelPVariant=InternalParameters  IdealPVariant=Disabled  IVariant=InternalParameters  DVariant=Disabled  IntegratorVariant=Discrete  SatVariant=Enabled  AWVariant=DiscClampingParallel  PCopyVariant=Disabled  TRVariant=Disabled  FdbkBlocksVariant=Forward  IdealPFdbkVariant=Disabled  SatFdbkVariant=Disabled  DerivativeFilterVariant=Disabled  NVariant=Disabled  NCopyVariant=Disabled_SignalSpec  FilterICVariant=Disabled  IntegratorICVariant=InternalICs  ExternalResetVariant=Disabled  TRSumVariant=Passthrough  SumFdbkVariant=Disabled  SumVariant=Sum_PI  TsampFilterVariant=InternalTs  TsampNgainVariant=Passthrough  TsampIntegralVariant=Disabled_SignalSpec  ExternalSaturationOutDataTypeStr=Inherit: Same as second input  DerivativeSourceVariant=Disabled  PreIntVariant=InternalPreInt
  Park1 : MATLAB Function  TreatAsAtomicUnit=on
  Park2 : MATLAB Function  TreatAsAtomicUnit=on
  Rad to deg1 : Gain  Gain=180/pi
  Rad to deg2 : Gain  Gain=180/pi
  RevPark1 : MATLAB Function  TreatAsAtomicUnit=on
  RevPark2 : MATLAB Function  TreatAsAtomicUnit=on
  Scope{10,15,17,19,29..30,34..36} (9 alike) : Scope  NumInputPorts=2
      Scope10 settings: ActiveDisplayYMinimum=-5.2481835137744008  ActiveDisplayYMaximum=47.233651623969614  DataLoggingVariableName=ScopeData27
      Scope15 settings: ActiveDisplayYMinimum=0.0075000000000000006  ActiveDisplayYMaximum=0.0325  DataLoggingVariableName=ScopeData34
      Scope17 settings: ActiveDisplayYMinimum=1363.1836491868808  ActiveDisplayYMaximum=1375.04702581976  DataLoggingVariableName=ScopeData36
      Scope19 settings: ActiveDisplayYMinimum=-9.7785388194430141  ActiveDisplayYMaximum=52.407441398347267  DataLoggingVariableName=ScopeData38
      Scope29 settings: ActiveDisplayYMinimum=-0.018504547079538081  ActiveDisplayYMaximum=0.49853620070628168  DataLoggingVariableName=ScopeData28
      Scope30 settings: ActiveDisplayYMinimum=-0.068250226127922337  ActiveDisplayYMaximum=0.064256506451961737  DataLoggingVariableName=ScopeData29
      Scope34 settings: ActiveDisplayYMinimum=-10.860061692792559  ActiveDisplayYMaximum=61.442988659524922  DataLoggingVariableName=ScopeData49
      Scope35 settings: ActiveDisplayYMinimum=-0.018504547079538081  ActiveDisplayYMaximum=0.49853620070628168  DataLoggingVariableName=ScopeData50
      Scope36 settings: ActiveDisplayYMinimum=-0.068250226127922337  ActiveDisplayYMaximum=0.064256506451961737  DataLoggingVariableName=ScopeData51
  Scope{11..12,16,18,21..28,31..33} (15 alike) : Scope
      Scope11 settings: ActiveDisplayYMinimum=-19.096901402816375  ActiveDisplayYMaximum=19.120590576315788  DataLoggingVariableName=ScopeData30
      Scope12 settings: ActiveDisplayYMinimum=0.0055558714492785766  ActiveDisplayYMaximum=0.04791549784383016  DataLoggingVariableName=ScopeData31
      Scope16 settings: ActiveDisplayYMinimum=-0.00045623090907525666  ActiveDisplayYMaximum=0.00044225246132360179  DataLoggingVariableName=ScopeData35
      Scope18 settings: ActiveDisplayYMinimum=-19.096901402816375  ActiveDisplayYMaximum=19.120590576315788  DataLoggingVariableName=ScopeData37
      Scope21 settings: ActiveDisplayYMinimum=-9.08103109878298  ActiveDisplayYMaximum=1.6684669955642857  DataLoggingVariableName=ScopeData40
      Scope22 settings: ActiveDisplayYMinimum=-70.559876705932709  ActiveDisplayYMaximum=631.53921004933659  DataLoggingVariableName=ScopeData41
      Scope23 settings: ActiveDisplayYMinimum=-1.5635296954169715  ActiveDisplayYMaximum=0.72593411203052016  DataLoggingVariableName=ScopeData42
      Scope24 settings: ActiveDisplayYMinimum=-0.0062150346375224163  ActiveDisplayYMaximum=0.055935311737701762  DataLoggingVariableName=ScopeData43
      Scope25 settings: ActiveDisplayYMinimum=-70.559876705932709  ActiveDisplayYMaximum=631.53921004933659  DataLoggingVariableName=ScopeData44
      Scope26 settings: ActiveDisplayYMinimum=-452.6835395386438  ActiveDisplayYMaximum=318.93705127381384  DataLoggingVariableName=ScopeData45
      Scope27 settings: ActiveDisplayYMinimum=-0.40449771436693455  ActiveDisplayYMaximum=0.64067173662257559  DataLoggingVariableName=ScopeData25
      Scope28 settings: ActiveDisplayYMinimum=-0.046646220623980633  ActiveDisplayYMaximum=0.10063848186154864  DataLoggingVariableName=ScopeData26
      Scope31 settings: ActiveDisplayYMinimum=-115.17645332437448  ActiveDisplayYMaximum=118.37044346456712  DataLoggingVariableName=ScopeData46
      Scope32 settings: ActiveDisplayYMinimum=-0.40449771436693455  ActiveDisplayYMaximum=0.64067173662257559  DataLoggingVariableName=ScopeData47
      Scope33 settings: ActiveDisplayYMinimum=-0.046646220623980633  ActiveDisplayYMaximum=0.10063848186154864  DataLoggingVariableName=ScopeData48
  Scope13 : Scope  NumInputPorts=4
      settings: ActiveDisplayYMinimum=-0.68813129304418319  ActiveDisplayYMaximum=6.2555990509558841  DataLoggingVariableName=ScopeData32
  Scope14 : Scope  NumInputPorts=3
      settings: ActiveDisplayYMinimum=-0.052783691584462819  ActiveDisplayYMaximum=0.4750532242601655  DataLoggingVariableName=ScopeData33
  Scope20 : Scope  NumInputPorts=4
      settings: ActiveDisplayYMinimum=-0.68813129304418319  ActiveDisplayYMaximum=6.2555990509558841  DataLoggingVariableName=ScopeData39
  Step : Step  Time=0  Before=0.01  After=0.01  SampleTime=0
  Step10 : Step  Time=0  Before=0.00544  After=0.00544  SampleTime=0
  Step11 : Step  Time=0  Before=0.0015  After=0.0015  SampleTime=0
  Step4 : Step  Time=0  Before=4.85  After=4.85  SampleTime=0
  Step5 : Step  Time=0  Before=0.00544  After=0.00544  SampleTime=0
  Step6 : Step  Time=0  Before=0.0015  After=0.0015  SampleTime=0
  Step8 : Step  Time=0  Before=0.01  After=0.01  SampleTime=0
  Step9 : Step  Time=0  Before=4.85  After=4.85  SampleTime=0
  Sum{,1..2,5..8} (7 alike) : Sum  Inputs=|+-
  Theta_elec1 : Gain  Gain=50
  Theta_elec2 : Gain  Gain=50
  减速器角度输出1 : Scope
      settings: ActiveDisplayYMinimum=-3.2575204385667078  ActiveDisplayYMaximum=25.318176358378867  DataLoggingVariableName=ScopeData53
  减速器角度输出2 : Scope
      settings: ActiveDisplayYMinimum=-3.2575204385667078  ActiveDisplayYMaximum=25.318176358378867  DataLoggingVariableName=ScopeData56
  减速器角速度输出1 : Scope
      settings: ActiveDisplayYMinimum=-0.049701649268213327  ActiveDisplayYMaximum=0.44324985732957672  DataLoggingVariableName=ScopeData54
  减速器角速度输出2 : Scope
      settings: ActiveDisplayYMinimum=-0.049701649268213327  ActiveDisplayYMaximum=0.44324985732957672  DataLoggingVariableName=ScopeData57
  D_Theta 4 : Outport
  D_w 4 : Outport  Port=2
  P_Theta 4 : Outport  Port=3
  P_w 4 : Outport  Port=4
  wires:
  Sum8/1 -> Scope23/1
  Sum1/1 -> Scope21/1
  Step8/1 -> Scope24/1, Motor2/1(TL)  "TL"
  Motor2/1(Vp) -> Scope18/1  "Vp"
  Motor2/2(Ip) -> Demux2/1, Scope27/1  "Ip"
  Park2/2(Iq) -> Scope20/3, Scope29/2, Sum7/2  "Iq"
  Park2/1(Id) -> Scope20/4, Scope30/2, Sum2/2  "Id"
  Constant11/1 -> Scope30/1, Sum2/1
  PID Controller6/1 -> Add2/1
  MATLAB Function4/1(I_mag) -> Scope29/1, Sum7/1
  Demux2/1 -> Park2/1(Ia)
  Sum7/1 -> PID Controller6/1
  Motor2/5(theta) -> MATLAB Function4/2(pos_real_rad), Rad to deg2/1, Theta_elec2/1  "theta"
  Constant12/1 -> MATLAB Function4/5(kp)
  Sum2/1 -> PID Controller5/1
  Step10/1 -> Motor2/3(L_in)
  Ke2/1 -> Add2/2
  Motor2/3(Te) -> Scope28/1  "Te"
  RevPark2/2(Vb_raw) -> Controlled Voltage Source6/1
  Step11/1 -> Motor2/4(psi_in)
  Theta_elec2/1 -> RevPark2/3(Theta_elec), Park2/3(Theta_elec)
  Constant17/1 -> MATLAB Function4/7(ki)
  Add2/1 -> Scope20/1, RevPark2/1(Vq)  "Vq_cmd"
  PID Controller5/1 -> Scope20/2, RevPark2/2(Vd)  "Vd_cmd"
  Step/1 -> Sum/2, Scope15/1, Motor1/1(TL)  "TL"
  Motor2/4(w) -> MATLAB Function4/4(vel_real_rads), Mini08-2/2(w), Sum8/2, Scope19/1, Ke2/1, Scope26/1  "w"
  MATLAB Function3/1(TL_est) -> Sum/1, Scope15/2, [TL], Scope12/1  "TL_est"
  Sum/1 -> Scope16/1
  PID Controller3/1 -> Scope13/2, RevPark1/2(Vd)  "Vd_cmd"
  Motor1/4(w) -> MATLAB Function2/4(vel_real_rads), Sum8/1, Scope19/2, Scope14/2, MATLAB Function3/2(wm), Ke1/1, Mini08-1/2(w), Scope31/1  "w"
  Step9/1 -> Motor2/2(IR_in)
  Add1/1 -> Scope13/1, RevPark1/1(Vq)  "Vq_cmd"
  Constant14/1 -> MATLAB Function2/5(kp)
  Park1/1(Id) -> Scope13/4, Scope36/2, Sum5/2  "Id"
  Constant6/1 -> MATLAB Function2/6(kv)
  Constant15/1 -> MATLAB Function4/6(kv)
  Constant7/1 -> MATLAB Function2/7(ki)
  Theta_elec1/1 -> RevPark1/3(Theta_elec), Park1/3(Theta_elec)
  Motor1/5(theta) -> Scope34/2, MATLAB Function2/2(pos_real_rad), Scope14/3, MATLAB Function3/3(theta_m), Rad to deg1/1, Theta_elec1/1  "theta"
  Sum5/1 -> PID Controller3/1
  Step5/1 -> Motor1/3(L_in)
  Ke1/1 -> Add1/2
  Step6/1 -> Motor1/4(psi_in)
  Sum6/1 -> PID Controller4/1
  Rad to deg1/1 -> Sum1/1, Scope17/2, Mini08-1/1(In2), Scope22/1  "Theta (degrees)"
  RevPark1/2(Vb_raw) -> Controlled Voltage Source4/1
  Demux2/2 -> Park2/2(Ib)
  Motor1/3(Te) -> Scope33/1  "Te"
  Rad to deg2/1 -> Sum1/2, Scope17/1, Mini08-2/1(In2), Scope25/1  "Theta (degrees)"
  RevPark1/1(Va_raw) -> Controlled Voltage Source3/1
  Constant8/1 -> MATLAB Function2/8(kd)
  Demux1/1 -> Park1/1(Ia)
  Motor1/1(Vp) -> Scope11/1  "Vp"
  RevPark2/1(Va_raw) -> Controlled Voltage Source5/1
  Step4/1 -> Motor1/2(IR_in)
  Park1/2(Iq) -> Scope13/3, Scope14/1, MATLAB Function3/1(iq), Scope35/2, Sum6/2  "Iq"
  Constant10/1 -> MATLAB Function4/8(kd)
  MATLAB Function2/1(I_mag) -> Scope35/1, Sum6/1
  Motor1/2(Ip) -> Demux1/1, Scope32/1  "Ip"
  Constant13/1 -> Scope36/1, Sum5/1
  PID Controller4/1 -> Add1/1
  Demux1/2 -> Park1/2(Ib)
  vel_ref4/1 -> Gain5/1
  Gain4/1 -> Scope10/1, Scope34/1, MATLAB Function2/1(pos_ref_rad), MATLAB Function4/1(pos_ref_rad)
  pos_ref4/1 -> Gain4/1
  Gain5/1 -> Scope10/2, MATLAB Function2/3(vel_ref_rads), MATLAB Function4/3(vel_ref_rads)
  Mini08-2/1("Theta ") -> D_Theta 4/1, 减速器角度输出1/1
  Mini08-2/2("w ") -> D_w 4/1, 减速器角速度输出1/1
  Mini08-1/2("w ") -> P_w 4/1, 减速器角速度输出2/1
  Mini08-1/1("Theta ") -> P_Theta 4/1, 减速器角度输出2/1
  connections:
  Motor1/LConn4 -- Controlled Voltage Source4/LConn1
  Motor2/LConn4 -- Controlled Voltage Source6/LConn1
  Motor1/LConn2 -- Controlled Voltage Source3/LConn1
  Motor2/LConn1 -- Controlled Voltage Source5/RConn1
  Motor1/LConn1 -- Controlled Voltage Source3/RConn1
  Motor2/LConn2 -- Controlled Voltage Source5/LConn1
  Motor1/LConn3 -- Controlled Voltage Source4/RConn1
  Motor2/LConn3 -- Controlled Voltage Source6/RConn1
